simulink model "simulinkExample"  (R2018b)
settings: Solver=FixedStepAuto  StartTime=0.0  StopTime=1  RelTol=1e-3
undefined symbols (not defined in the file): f
libraries: instrumentlib x2
settings Model: Creator=drone1  LastModifiedBy=dskaputa
settings DebuggingCC: LibraryContextMissingDiagnostic=none
settings SFSimCC: SimUseLocalCustomCode=off
settings RTWCC: RTWUseLocalCustomCode=off

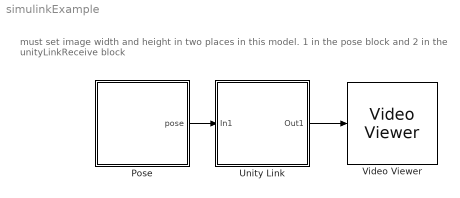
== system simulinkExample ==
  note: must set image width and height in two places in this model. 1 in the pose block and 2 in the unityLinkReceive block
  Pose : Subsystem
  Unity Link : Subsystem  Priority=2
      mask Display: image('unity.png');
  Video Viewer : VideoViewer  Priority=3  FigPos=[-749.4 779.6 557.6 424.8]
  wires:
  Pose/1(pose) -> Unity Link/1(In1)
  Unity Link/1(Out1) -> Video Viewer/1

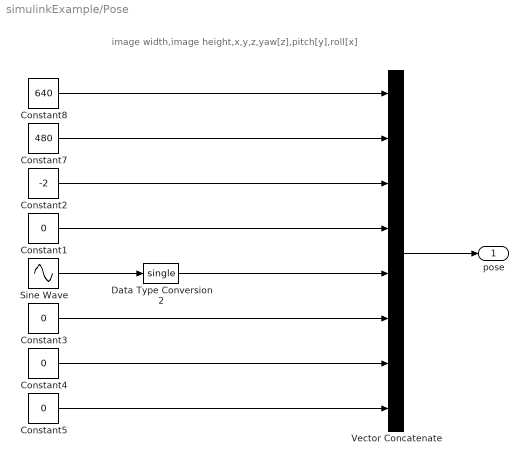
== system simulinkExample/Pose ==
  note: image width,image height,x,y,z,yaw[z],pitch[y],roll[x]
  Constant{1,3..5} (4 alike) : Constant  Value=0  OutDataTypeStr=single
  Constant2 : Constant  Value=-2  OutDataTypeStr=single
  Constant7 : Constant  Value=480  OutDataTypeStr=single
  Constant8 : Constant  Value=640  OutDataTypeStr=single
  Data Type Conversion2 : DataTypeConversion  OutDataTypeStr=single
  Sine Wave : Sin  SampleTime=0.01
  Vector Concatenate : Concatenate  NumInputs=8
  pose : Outport
  wires:
  Vector Concatenate/1 -> pose/1
  Sine Wave/1 -> Data Type Conversion2/1
  Constant5/1 -> Vector Concatenate/8
  Constant4/1 -> Vector Concatenate/7
  Constant3/1 -> Vector Concatenate/6
  Data Type Conversion2/1 -> Vector Concatenate/5
  Constant1/1 -> Vector Concatenate/4
  Constant2/1 -> Vector Concatenate/3
  Constant7/1 -> Vector Concatenate/2
  Constant8/1 -> Vector Concatenate/1

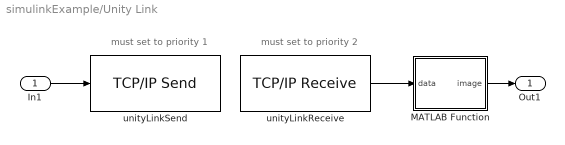
== system simulinkExample/Unity Link ==
  note: must set to priority 1
  note: must set to priority 2
  In1 : Inport
  MATLAB Function : MATLAB Function  TreatAsAtomicUnit=on
  "unityLinkReceive " : instrumentlib/TCP//IP Receive  Priority=2  Host=127.0.0.1  Port=55001  DataSize="[640  480    3]"  EnableBlockingMode=on  Timeout=20  SampleTime=-1  DataType=uint8  ByteOrder=LittleEndian  ASCIIFormatting=%f,  Terminator=LF
      settings: SourceProductName=Instrument Control Toolbox
  "unityLinkSend " : instrumentlib/TCP//IP Send  Priority=1  Host=127.0.0.1  Port=55001  EnableBlockingMode=on  Timeout=10  ByteOrder=LittleEndian  TransferDelay=off
      settings: SourceProductName=Instrument Control Toolbox
  Out1 : Outport
  wires:
  "unityLinkReceive "/1 -> MATLAB Function/1(data)
  In1/1 -> "unityLinkSend "/1
  MATLAB Function/1(image) -> Out1/1

== matlab function simulinkExample/Unity Link/MATLAB Function ==
  data: data input; image output
function image = fcn(data)
x = size(data);
width = x(1);
height = x(2);
temp = reshape(data,[3,width*height]);
image = imrotate(reshape(temp',[width,height,3]),90);
